simulink model "BrownZhangControl"  (R2017a)
settings: Solver=FixedStepAuto  StartTime=0.0  StopTime=10  FixedStep=0.001  RelTol=1e-3
InitFcn:
  | Kf = 0.01;
  | Ke = 0.001;
  | 
  | global w;
  | w =200;
  | % actual == 377
  | 
  | % w = 200; % estimate in rad/s
undefined symbols (not defined in the file or in its folder): DiscIntNeverNeededParam
settings Model: Creator=djorna  LastModifiedBy=djorna

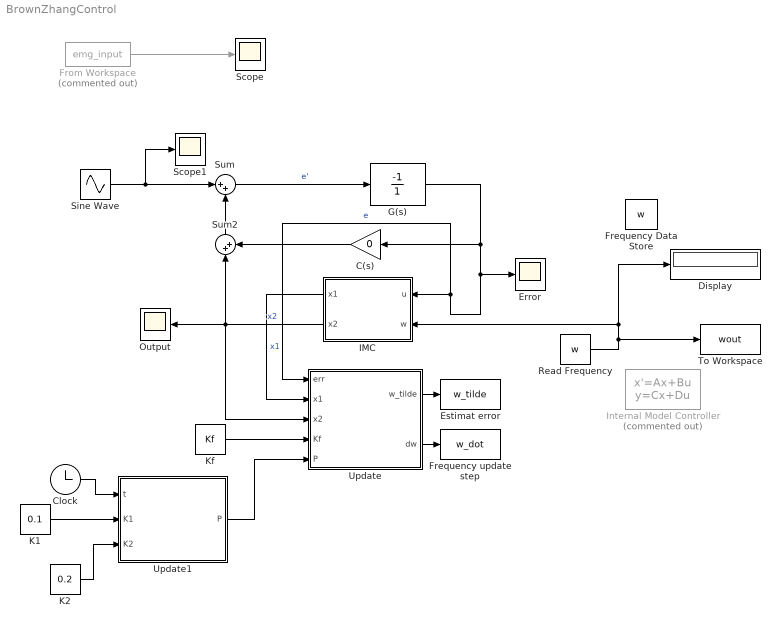
== system BrownZhangControl ==
  C(s) : Gain  Gain=0
  Clock : Clock
      settings: Decimation=1000
  Display : Display
  Error : Scope
  Estimat error : ToWorkspace  VariableName=w_tilde  SaveFormat=Timeseries  SampleTime=-1
  Frequency Data Store : DataStoreMemory  DataStoreName=w  ReadBeforeWriteMsg=warning  WriteAfterWriteMsg=warning  WriteAfterReadMsg=warning  InitialValue=200  ShowAdditionalParam=off  OutDataTypeStr=double
  Frequency update step : ToWorkspace  VariableName=w_dot  SaveFormat=Timeseries  SampleTime=-1
  From Workspace : FromWorkspace  Commented=on  VariableName=emg_input  SampleTime=1/2000
  G(s) : TransferFcn  Numerator=-1  Denominator=[1]
  IMC : Subsystem
  Internal Model Controller : StateSpace  Commented=on  A=[0 w; -w 0]  B=[0; Kf]  C=[1 0; 0 1]  D=[0; 0]  X0=0  ContinuousStateAttributes='frequency'
  K1 : Constant  Value=0.1
  K2 : Constant  Value=0.2
  Kf : Constant  Value=Kf
  Output : Scope
  Read Frequency : DataStoreRead  DataStoreName=w
  Scope : Scope
  Scope1 : Scope
  Sine Wave : Sin  Frequency=500  SampleTime=0
  Sum : Sum  Inputs=|++
  Sum2 : Sum  Inputs=|++
  To Workspace : ToWorkspace  VariableName=wout  SaveFormat=Timeseries  SampleTime=-1
  Update : MATLAB Function  TreatAsAtomicUnit=on
  Update1 : MATLAB Function  TreatAsAtomicUnit=on
  wires:
  Sum/1 -> G(s)/1  "e'"
  G(s)/1 -> IMC/1(u), Update/1(err), Error/1, C(s)/1  "e"
  C(s)/1 -> Sum2/2
  Sum2/1 -> Sum/2
  From Workspace/1 -> Scope/1
  Sine Wave/1 -> Scope1/1, Sum/1
  Kf/1 -> Update/4(Kf)
  Update/1(w_tilde) -> Estimat error/1
  Update/2(dw) -> Frequency update step/1
  IMC/1(x1) -> Update/2(x1)  "x1"
  IMC/2(x2) -> Update/3(x2), Output/1, Sum2/1  "x2"
  K2/1 -> Update1/3(K2)
  K1/1 -> Update1/2(K1)
  Clock/1 -> Update1/1(t)
  Update1/1(P) -> Update/5(P)
  Read Frequency/1 -> IMC/2(w), Display/1, To Workspace/1

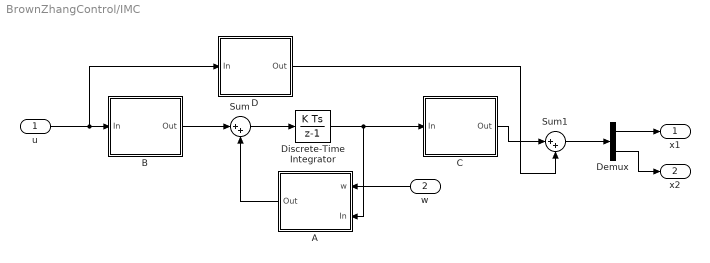
== system BrownZhangControl/IMC ==
  u : Inport  PortDimensions=1
  w : Inport  Port=2
  A : Subsystem
  B : Subsystem
  C : Subsystem
  D : Subsystem
  Demux : Demux  Outputs=2
  Discrete-Time Integrator : DiscreteIntegrator  InitialConditionSetting=State (most efficient)  SampleTime=-1  ICPrevOutput=DiscIntNeverNeededParam  ICPrevScaledInput=DiscIntNeverNeededParam
  Sum : Sum  Inputs=|++
  Sum1 : Sum  Inputs=|++
  x1 : Outport
  x2 : Outport  Port=2
  wires:
  Demux/1 -> x1/1
  u/1 -> D/1(In), B/1(In)
  Demux/2 -> x2/1
  A/1(Out) -> Sum/2
  Sum/1 -> Discrete-Time Integrator/1
  Discrete-Time Integrator/1 -> C/1(In), A/2(In)
  w/1 -> A/1(w)
  B/1(Out) -> Sum/1
  C/1(Out) -> Sum1/1
  D/1(Out) -> Sum1/2
  Sum1/1 -> Demux/1

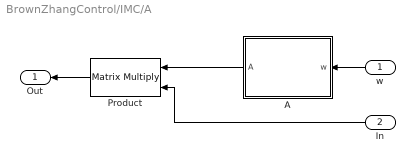
== system BrownZhangControl/IMC/A ==
  w : Inport
  In : Inport  Port=2  PortDimensions=[2 1]
  A : MATLAB Function  TreatAsAtomicUnit=on
  Product : Product  Multiplication=Matrix(*)
  Out : Outport
  wires:
  A/1(A) -> Product/1
  In/1 -> Product/2
  Product/1 -> Out/1
  w/1 -> A/1(w)

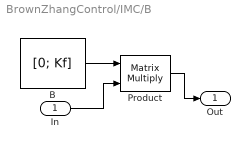
== system BrownZhangControl/IMC/B ==
  In : Inport  PortDimensions=1
  B : Constant  Value=[0; Kf]
  Product : Product  Multiplication=Matrix(*)
  Out : Outport
  wires:
  B/1 -> Product/1
  Product/1 -> Out/1
  In/1 -> Product/2

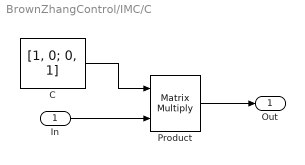
== system BrownZhangControl/IMC/C ==
  In : Inport
  C : Constant  Value=[1, 0; 0, 1]
  Product : Product  Multiplication=Matrix(*)
  Out : Outport  PortDimensions=[2 1]
  wires:
  C/1 -> Product/1
  Product/1 -> Out/1
  In/1 -> Product/2

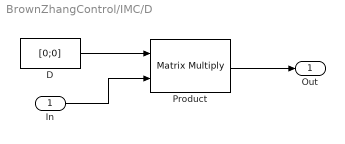
== system BrownZhangControl/IMC/D ==
  In : Inport
  D : Constant  Value=[0;0]
  Product : Product  Multiplication=Matrix(*)
  Out : Outport  PortDimensions=2
  wires:
  D/1 -> Product/1
  Product/1 -> Out/1
  In/1 -> Product/2

== matlab function BrownZhangControl/Update1 ==
  data: t input; P output; K1 input; K2 input
function P  = adapt_gain(t,K1, K2)
    P = K1 / (K2*t + 1);
end

== matlab function BrownZhangControl/Update ==
  data: w_tilde output; dw output; err input; x1 input; x2 input; Kf input; P input; w data_store_memory
function [w_tilde, dw] = update_w(err, x1, x2, Kf, P)
    global w;
    if isnan(w)
        w = 200;
    end
    w_tilde = - (w * Kf * err * x1) / ((w*x1)^2 + x2^2);
    dw = P * w_tilde;
    w = w + dw;    
end

== matlab function BrownZhangControl/IMC/A/A ==
  data: w input; A output
function A = A_Mat(w)
A = [0 w; -w 0];
